simulink model "Quanser_AERO_Simulation_2020b"  (R2020b)
settings: Solver=ode45  StartTime=0.0  StopTime=sim_time  FixedStep=0.01  RelTol=1e-3
InitFcn:
  | % Run simulation parameters
  | quanser_AERO_sim_params;
model workspace (MAT data in the model file):
  a : Simulink.Parameter (value not decoded)
  a_a : Simulink.Parameter (value not decoded)
  b : Simulink.Parameter (value not decoded)
  b_b : Simulink.Parameter (value not decoded)
  c : Simulink.Parameter (value not decoded)
  c_c : Simulink.Parameter (value not decoded)
  d : Simulink.Parameter (value not decoded)
  d_d : Simulink.Parameter (value not decoded)
  e : Simulink.Parameter (value not decoded)
  f : Simulink.Parameter (value not decoded)
  g : Simulink.Parameter (value not decoded)
  p_p : Simulink.Parameter (value not decoded)
  smiData : object (value not decoded)
  t_t : Simulink.Parameter (value not decoded)
  u_lim : Simulink.Parameter (value not decoded)
  y_y : Simulink.Parameter (value not decoded)
  z_z : Simulink.Parameter (value not decoded)
values from neighbouring files (symbols this model uses):
  model = 2    [quanser_AERO_sim_params.m]
  ts = 0.002    [quanser_AERO_sim_params.m]
symbols that are objects in the model workspace (value not decoded): a, a_a, b, b_b, c, c_c, d, d_d, f, g, p_p, smiData, t_t, u_lim, y_y, z_z
undefined symbols (not defined in the file or in its folder): A, B, C, den1, den2, ini_cond, K, K_D1, K_D2, K_I1, K_I2, K_P1, K_P2, KI, KX, L, Nbar, noise, num1, num2, tau_p, X, Y, Z
libraries: sm_lib x175, nesl_utility x35, simulink x31
(part 5 of 5)

== system Quanser_AERO_Simulation_2020b/Quanser AERO3/Digital Twin/AERO_Base1_RIGID ==
  ReferenceFrame : sm_lib/Frames and Transforms/Reference Frame
  Solid : sm_lib/Body Elements/File Solid  ExtGeomFileName=AERO - Base_ipt_b1761deb.STEP  UnitType=FromFile  ExtGeomFileUnits=m  StepReaderType=HEX  ExportConvexHullGeometry=off  InertiaType=Custom  Mass=smiData.Solid(1).mass  MassUnits=kg  CenterOfMass=smiData.Solid(1).CoM  CenterOfMassUnits=mm  MomentsOfInertia=smiData.Solid(1).MoI  MomentsOfInertiaUnits=kg*mm^2  ProductsOfInertia=smiData.Solid(1).PoI  ProductsOfInertiaUnits=kg*mm^2  BasedOnType=DensityFromFile  Density=1000  DensityUnits=kg/m^3  DoExposeReferenceFrame=on  SerializedFrames=<Frames/>  GraphicType=FromGeometry  MarkerShape=Sphere  MarkerSize=10  GraphicVisPropType=SimpleVisualProperties  GraphicDiffuseColor=smiData.Solid(1).color  GraphicSpecularColor=[0.5 0.5 0.5 1.0]  GraphicAmbientColor=[0.15 0.15 0.15 1.0]  GraphicEmissiveColor=[0.0 0.0 0.0 1.0]  GraphicShininess=75  GraphicOpacity=smiData.Solid(1).opacity
  Transform : sm_lib/Frames and Transforms/Rigid Transform  TranslationMethod=Cartesian  TranslationStandardOffset=0  TranslationLengthUnit=mm  TranslationStandardAxis=+Z  TranslationCartesianOffset=smiData.RigidTransform(7).translation  TranslationROffset=0  TranslationROffsetUnits=m  TranslationZOffset=0  TranslationZOffsetUnits=m  TranslationThetaOffset=0  TranslationThetaOffsetUnits=deg  RotationMethod=ArbitraryAxis  RotationAngleUnits=rad  RotationStandardAxis=+Z  RotationAngle=smiData.RigidTransform(7).angle  RotationArbitraryAxis=smiData.RigidTransform(7).axis  FollAlignAxisA=+X  BaseAlignAxisA=+Y  FollAlignAxisB=+Y  BaseAlignAxisB=+Z  RotationSequenceAxes=FollowerAxes  RotationSequence=XYX  RotationSequenceAngles=[0 0 0]  RotationSequenceAnglesUnits=deg  RotationMatrix=[1 0 0; 0 1 0; 0 0 1]
  F1 : PMIOPort  Side=Left
  F : PMIOPort  Port=2  Side=Right
  connections:
  ReferenceFrame/RConn1 -- Solid/RConn1 -- Transform/LConn1 -- F1/RConn1
  Transform/RConn1 -- F/RConn1

== system Quanser_AERO_Simulation_2020b/Quanser AERO3/Digital Twin/AERO_Fork1_RIGID ==
  ReferenceFrame : sm_lib/Frames and Transforms/Reference Frame
  Solid : sm_lib/Body Elements/File Solid  ExtGeomFileName=AERO - Fork_ipt_cc713931.STEP  UnitType=FromFile  ExtGeomFileUnits=m  StepReaderType=HEX  ExportConvexHullGeometry=off  InertiaType=Custom  Mass=smiData.Solid(2).mass  MassUnits=kg  CenterOfMass=smiData.Solid(2).CoM  CenterOfMassUnits=mm  MomentsOfInertia=smiData.Solid(2).MoI  MomentsOfInertiaUnits=kg*mm^2  ProductsOfInertia=smiData.Solid(2).PoI  ProductsOfInertiaUnits=kg*mm^2  BasedOnType=DensityFromFile  Density=1000  DensityUnits=kg/m^3  DoExposeReferenceFrame=on  SerializedFrames=<Frames/>  GraphicType=FromGeometry  MarkerShape=Sphere  MarkerSize=10  GraphicVisPropType=SimpleVisualProperties  GraphicDiffuseColor=smiData.Solid(2).color  GraphicSpecularColor=[0.5 0.5 0.5 1.0]  GraphicAmbientColor=[0.15 0.15 0.15 1.0]  GraphicEmissiveColor=[0.0 0.0 0.0 1.0]  GraphicShininess=75  GraphicOpacity=smiData.Solid(2).opacity
  Transform : sm_lib/Frames and Transforms/Rigid Transform  TranslationMethod=Cartesian  TranslationStandardOffset=0  TranslationLengthUnit=mm  TranslationStandardAxis=+Z  TranslationCartesianOffset=smiData.RigidTransform(1).translation  TranslationROffset=0  TranslationROffsetUnits=m  TranslationZOffset=0  TranslationZOffsetUnits=m  TranslationThetaOffset=0  TranslationThetaOffsetUnits=deg  RotationMethod=ArbitraryAxis  RotationAngleUnits=rad  RotationStandardAxis=+Z  RotationAngle=smiData.RigidTransform(1).angle  RotationArbitraryAxis=smiData.RigidTransform(1).axis  FollAlignAxisA=+X  BaseAlignAxisA=+Y  FollAlignAxisB=+Y  BaseAlignAxisB=+Z  RotationSequenceAxes=FollowerAxes  RotationSequence=XYX  RotationSequenceAngles=[0 0 0]  RotationSequenceAnglesUnits=deg  RotationMatrix=[1 0 0; 0 1 0; 0 0 1]
  Transform1 : sm_lib/Frames and Transforms/Rigid Transform  TranslationMethod=Cartesian  TranslationStandardOffset=0  TranslationLengthUnit=mm  TranslationStandardAxis=+Z  TranslationCartesianOffset=smiData.RigidTransform(8).translation  TranslationROffset=0  TranslationROffsetUnits=m  TranslationZOffset=0  TranslationZOffsetUnits=m  TranslationThetaOffset=0  TranslationThetaOffsetUnits=deg  RotationMethod=ArbitraryAxis  RotationAngleUnits=rad  RotationStandardAxis=+Z  RotationAngle=smiData.RigidTransform(8).angle  RotationArbitraryAxis=smiData.RigidTransform(8).axis  FollAlignAxisA=+X  BaseAlignAxisA=+Y  FollAlignAxisB=+Y  BaseAlignAxisB=+Z  RotationSequenceAxes=FollowerAxes  RotationSequence=XYX  RotationSequenceAngles=[0 0 0]  RotationSequenceAnglesUnits=deg  RotationMatrix=[1 0 0; 0 1 0; 0 0 1]
  F1 : PMIOPort  Side=Left
  F : PMIOPort  Port=2  Side=Right
  connections:
  Transform/LConn1 -- Transform1/LConn1 -- ReferenceFrame/RConn1 -- Solid/RConn1
  Transform/RConn1 -- F/RConn1
  Transform1/RConn1 -- F1/RConn1

== system Quanser_AERO_Simulation_2020b/Quanser AERO3/Digital Twin/AERO_Propeller1_RIGID ==
  ReferenceFrame : sm_lib/Frames and Transforms/Reference Frame
  Solid : sm_lib/Body Elements/File Solid  ExtGeomFileName=AERO - Propeller_ipt_36a575e7.STEP  UnitType=FromFile  ExtGeomFileUnits=m  StepReaderType=HEX  ExportConvexHullGeometry=off  InertiaType=Custom  Mass=smiData.Solid(5).mass  MassUnits=kg  CenterOfMass=smiData.Solid(5).CoM  CenterOfMassUnits=mm  MomentsOfInertia=smiData.Solid(5).MoI  MomentsOfInertiaUnits=kg*mm^2  ProductsOfInertia=smiData.Solid(5).PoI  ProductsOfInertiaUnits=kg*mm^2  BasedOnType=DensityFromFile  Density=1000  DensityUnits=kg/m^3  DoExposeReferenceFrame=on  SerializedFrames=<Frames/>  GraphicType=FromGeometry  MarkerShape=Sphere  MarkerSize=10  GraphicVisPropType=SimpleVisualProperties  GraphicDiffuseColor=smiData.Solid(5).color  GraphicSpecularColor=[0.5 0.5 0.5 1.0]  GraphicAmbientColor=[0.15 0.15 0.15 1.0]  GraphicEmissiveColor=[0.0 0.0 0.0 1.0]  GraphicShininess=75  GraphicOpacity=smiData.Solid(5).opacity
  Transform : sm_lib/Frames and Transforms/Rigid Transform  TranslationMethod=Cartesian  TranslationStandardOffset=0  TranslationLengthUnit=mm  TranslationStandardAxis=+Z  TranslationCartesianOffset=smiData.RigidTransform(10).translation  TranslationROffset=0  TranslationROffsetUnits=m  TranslationZOffset=0  TranslationZOffsetUnits=m  TranslationThetaOffset=0  TranslationThetaOffsetUnits=deg  RotationMethod=ArbitraryAxis  RotationAngleUnits=rad  RotationStandardAxis=+Z  RotationAngle=smiData.RigidTransform(10).angle  RotationArbitraryAxis=smiData.RigidTransform(10).axis  FollAlignAxisA=+X  BaseAlignAxisA=+Y  FollAlignAxisB=+Y  BaseAlignAxisB=+Z  RotationSequenceAxes=FollowerAxes  RotationSequence=XYX  RotationSequenceAngles=[0 0 0]  RotationSequenceAnglesUnits=deg  RotationMatrix=[1 0 0; 0 1 0; 0 0 1]
  F : PMIOPort  Side=Left
  connections:
  ReferenceFrame/RConn1 -- Solid/RConn1 -- Transform/LConn1
  Transform/RConn1 -- F/RConn1

== system Quanser_AERO_Simulation_2020b/Quanser AERO3/Digital Twin/AERO_Propeller2_RIGID ==
  ReferenceFrame : sm_lib/Frames and Transforms/Reference Frame
  Solid : sm_lib/Body Elements/File Solid  ExtGeomFileName=AERO - Propeller_ipt_36a575e7.STEP  UnitType=FromFile  ExtGeomFileUnits=m  StepReaderType=HEX  ExportConvexHullGeometry=off  InertiaType=Custom  Mass=smiData.Solid(5).mass  MassUnits=kg  CenterOfMass=smiData.Solid(5).CoM  CenterOfMassUnits=mm  MomentsOfInertia=smiData.Solid(5).MoI  MomentsOfInertiaUnits=kg*mm^2  ProductsOfInertia=smiData.Solid(5).PoI  ProductsOfInertiaUnits=kg*mm^2  BasedOnType=DensityFromFile  Density=1000  DensityUnits=kg/m^3  DoExposeReferenceFrame=on  SerializedFrames=<Frames/>  GraphicType=FromGeometry  MarkerShape=Sphere  MarkerSize=10  GraphicVisPropType=SimpleVisualProperties  GraphicDiffuseColor=smiData.Solid(5).color  GraphicSpecularColor=[0.5 0.5 0.5 1.0]  GraphicAmbientColor=[0.15 0.15 0.15 1.0]  GraphicEmissiveColor=[0.0 0.0 0.0 1.0]  GraphicShininess=75  GraphicOpacity=smiData.Solid(5).opacity
  Transform : sm_lib/Frames and Transforms/Rigid Transform  TranslationMethod=Cartesian  TranslationStandardOffset=0  TranslationLengthUnit=mm  TranslationStandardAxis=+Z  TranslationCartesianOffset=smiData.RigidTransform(12).translation  TranslationROffset=0  TranslationROffsetUnits=m  TranslationZOffset=0  TranslationZOffsetUnits=m  TranslationThetaOffset=0  TranslationThetaOffsetUnits=deg  RotationMethod=ArbitraryAxis  RotationAngleUnits=rad  RotationStandardAxis=+Z  RotationAngle=smiData.RigidTransform(12).angle  RotationArbitraryAxis=smiData.RigidTransform(12).axis  FollAlignAxisA=+X  BaseAlignAxisA=+Y  FollAlignAxisB=+Y  BaseAlignAxisB=+Z  RotationSequenceAxes=FollowerAxes  RotationSequence=XYX  RotationSequenceAngles=[0 0 0]  RotationSequenceAnglesUnits=deg  RotationMatrix=[1 0 0; 0 1 0; 0 0 1]
  F : PMIOPort  Side=Left
  connections:
  ReferenceFrame/RConn1 -- Solid/RConn1 -- Transform/LConn1
  Transform/RConn1 -- F/RConn1

== system Quanser_AERO_Simulation_2020b/Quanser AERO3/Digital Twin/AERO_Propeller_Housing1_RIGID ==
  ReferenceFrame : sm_lib/Frames and Transforms/Reference Frame
  Solid : sm_lib/Body Elements/File Solid  ExtGeomFileName=AERO - Propeller Housing_ipt_f68ac60a.STEP  UnitType=FromFile  ExtGeomFileUnits=m  StepReaderType=HEX  ExportConvexHullGeometry=off  InertiaType=Custom  Mass=smiData.Solid(4).mass  MassUnits=kg  CenterOfMass=smiData.Solid(4).CoM  CenterOfMassUnits=mm  MomentsOfInertia=smiData.Solid(4).MoI  MomentsOfInertiaUnits=kg*mm^2  ProductsOfInertia=smiData.Solid(4).PoI  ProductsOfInertiaUnits=kg*mm^2  BasedOnType=DensityFromFile  Density=1000  DensityUnits=kg/m^3  DoExposeReferenceFrame=on  SerializedFrames=<Frames/>  GraphicType=FromGeometry  MarkerShape=Sphere  MarkerSize=10  GraphicVisPropType=SimpleVisualProperties  GraphicDiffuseColor=smiData.Solid(4).color  GraphicSpecularColor=[0.5 0.5 0.5 1.0]  GraphicAmbientColor=[0.15 0.15 0.15 1.0]  GraphicEmissiveColor=[0.0 0.0 0.0 1.0]  GraphicShininess=75  GraphicOpacity=smiData.Solid(4).opacity
  Transform : sm_lib/Frames and Transforms/Rigid Transform  TranslationMethod=Cartesian  TranslationStandardOffset=0  TranslationLengthUnit=mm  TranslationStandardAxis=+Z  TranslationCartesianOffset=smiData.RigidTransform(4).translation  TranslationROffset=0  TranslationROffsetUnits=m  TranslationZOffset=0  TranslationZOffsetUnits=m  TranslationThetaOffset=0  TranslationThetaOffsetUnits=deg  RotationMethod=ArbitraryAxis  RotationAngleUnits=rad  RotationStandardAxis=+Z  RotationAngle=smiData.RigidTransform(4).angle  RotationArbitraryAxis=smiData.RigidTransform(4).axis  FollAlignAxisA=+X  BaseAlignAxisA=+Y  FollAlignAxisB=+Y  BaseAlignAxisB=+Z  RotationSequenceAxes=FollowerAxes  RotationSequence=XYX  RotationSequenceAngles=[0 0 0]  RotationSequenceAnglesUnits=deg  RotationMatrix=[1 0 0; 0 1 0; 0 0 1]
  Transform1 : sm_lib/Frames and Transforms/Rigid Transform  TranslationMethod=Cartesian  TranslationStandardOffset=0  TranslationLengthUnit=mm  TranslationStandardAxis=+Z  TranslationCartesianOffset=smiData.RigidTransform(9).translation  TranslationROffset=0  TranslationROffsetUnits=m  TranslationZOffset=0  TranslationZOffsetUnits=m  TranslationThetaOffset=0  TranslationThetaOffsetUnits=deg  RotationMethod=ArbitraryAxis  RotationAngleUnits=rad  RotationStandardAxis=+Z  RotationAngle=smiData.RigidTransform(9).angle  RotationArbitraryAxis=smiData.RigidTransform(9).axis  FollAlignAxisA=+X  BaseAlignAxisA=+Y  FollAlignAxisB=+Y  BaseAlignAxisB=+Z  RotationSequenceAxes=FollowerAxes  RotationSequence=XYX  RotationSequenceAngles=[0 0 0]  RotationSequenceAnglesUnits=deg  RotationMatrix=[1 0 0; 0 1 0; 0 0 1]
  F : PMIOPort  Side=Left
  F1 : PMIOPort  Port=2  Side=Right
  connections:
  ReferenceFrame/RConn1 -- Solid/RConn1 -- Transform/LConn1 -- Transform1/LConn1
  Transform/RConn1 -- F/RConn1
  Transform1/RConn1 -- F1/RConn1

== system Quanser_AERO_Simulation_2020b/Quanser AERO3/Digital Twin/AERO_Propeller_Housing2_RIGID ==
  ReferenceFrame : sm_lib/Frames and Transforms/Reference Frame
  Solid : sm_lib/Body Elements/File Solid  ExtGeomFileName=AERO - Propeller Housing_ipt_f68ac60a.STEP  UnitType=FromFile  ExtGeomFileUnits=m  StepReaderType=HEX  ExportConvexHullGeometry=off  InertiaType=Custom  Mass=smiData.Solid(4).mass  MassUnits=kg  CenterOfMass=smiData.Solid(4).CoM  CenterOfMassUnits=mm  MomentsOfInertia=smiData.Solid(4).MoI  MomentsOfInertiaUnits=kg*mm^2  ProductsOfInertia=smiData.Solid(4).PoI  ProductsOfInertiaUnits=kg*mm^2  BasedOnType=DensityFromFile  Density=1000  DensityUnits=kg/m^3  DoExposeReferenceFrame=on  SerializedFrames=<Frames/>  GraphicType=FromGeometry  MarkerShape=Sphere  MarkerSize=10  GraphicVisPropType=SimpleVisualProperties  GraphicDiffuseColor=smiData.Solid(4).color  GraphicSpecularColor=[0.5 0.5 0.5 1.0]  GraphicAmbientColor=[0.15 0.15 0.15 1.0]  GraphicEmissiveColor=[0.0 0.0 0.0 1.0]  GraphicShininess=75  GraphicOpacity=smiData.Solid(4).opacity
  Transform : sm_lib/Frames and Transforms/Rigid Transform  TranslationMethod=Cartesian  TranslationStandardOffset=0  TranslationLengthUnit=mm  TranslationStandardAxis=+Z  TranslationCartesianOffset=smiData.RigidTransform(6).translation  TranslationROffset=0  TranslationROffsetUnits=m  TranslationZOffset=0  TranslationZOffsetUnits=m  TranslationThetaOffset=0  TranslationThetaOffsetUnits=deg  RotationMethod=ArbitraryAxis  RotationAngleUnits=rad  RotationStandardAxis=+Z  RotationAngle=smiData.RigidTransform(6).angle  RotationArbitraryAxis=smiData.RigidTransform(6).axis  FollAlignAxisA=+X  BaseAlignAxisA=+Y  FollAlignAxisB=+Y  BaseAlignAxisB=+Z  RotationSequenceAxes=FollowerAxes  RotationSequence=XYX  RotationSequenceAngles=[0 0 0]  RotationSequenceAnglesUnits=deg  RotationMatrix=[1 0 0; 0 1 0; 0 0 1]
  Transform1 : sm_lib/Frames and Transforms/Rigid Transform  TranslationMethod=Cartesian  TranslationStandardOffset=0  TranslationLengthUnit=mm  TranslationStandardAxis=+Z  TranslationCartesianOffset=smiData.RigidTransform(11).translation  TranslationROffset=0  TranslationROffsetUnits=m  TranslationZOffset=0  TranslationZOffsetUnits=m  TranslationThetaOffset=0  TranslationThetaOffsetUnits=deg  RotationMethod=ArbitraryAxis  RotationAngleUnits=rad  RotationStandardAxis=+Z  RotationAngle=smiData.RigidTransform(11).angle  RotationArbitraryAxis=smiData.RigidTransform(11).axis  FollAlignAxisA=+X  BaseAlignAxisA=+Y  FollAlignAxisB=+Y  BaseAlignAxisB=+Z  RotationSequenceAxes=FollowerAxes  RotationSequence=XYX  RotationSequenceAngles=[0 0 0]  RotationSequenceAnglesUnits=deg  RotationMatrix=[1 0 0; 0 1 0; 0 0 1]
  F : PMIOPort  Side=Left
  F1 : PMIOPort  Port=2  Side=Right
  connections:
  ReferenceFrame/RConn1 -- Solid/RConn1 -- Transform/LConn1 -- Transform1/LConn1
  Transform/RConn1 -- F/RConn1
  Transform1/RConn1 -- F1/RConn1

== system Quanser_AERO_Simulation_2020b/Quanser AERO4/Digital Twin/AERO_Arm1_RIGID ==
  ReferenceFrame : sm_lib/Frames and Transforms/Reference Frame
  Solid : sm_lib/Body Elements/File Solid  ExtGeomFileName=AERO - Arm_ipt_54056d2d.STEP  UnitType=FromFile  ExtGeomFileUnits=m  StepReaderType=HEX  ExportConvexHullGeometry=off  InertiaType=Custom  Mass=smiData.Solid(3).mass  MassUnits=kg  CenterOfMass=smiData.Solid(3).CoM  CenterOfMassUnits=mm  MomentsOfInertia=smiData.Solid(3).MoI  MomentsOfInertiaUnits=kg*mm^2  ProductsOfInertia=smiData.Solid(3).PoI  ProductsOfInertiaUnits=kg*mm^2  BasedOnType=DensityFromFile  Density=1000  DensityUnits=kg/m^3  DoExposeReferenceFrame=on  SerializedFrames=<Frames/>  GraphicType=FromGeometry  MarkerShape=Sphere  MarkerSize=10  GraphicVisPropType=SimpleVisualProperties  GraphicDiffuseColor=smiData.Solid(3).color  GraphicSpecularColor=[0.5 0.5 0.5 1.0]  GraphicAmbientColor=[0.15 0.15 0.15 1.0]  GraphicEmissiveColor=[0.0 0.0 0.0 1.0]  GraphicShininess=75  GraphicOpacity=smiData.Solid(3).opacity
  Transform : sm_lib/Frames and Transforms/Rigid Transform  TranslationMethod=Cartesian  TranslationStandardOffset=0  TranslationLengthUnit=mm  TranslationStandardAxis=+Z  TranslationCartesianOffset=smiData.RigidTransform(2).translation  TranslationROffset=0  TranslationROffsetUnits=m  TranslationZOffset=0  TranslationZOffsetUnits=m  TranslationThetaOffset=0  TranslationThetaOffsetUnits=deg  RotationMethod=ArbitraryAxis  RotationAngleUnits=rad  RotationStandardAxis=+Z  RotationAngle=smiData.RigidTransform(2).angle  RotationArbitraryAxis=smiData.RigidTransform(2).axis  FollAlignAxisA=+X  BaseAlignAxisA=+Y  FollAlignAxisB=+Y  BaseAlignAxisB=+Z  RotationSequenceAxes=FollowerAxes  RotationSequence=XYX  RotationSequenceAngles=[0 0 0]  RotationSequenceAnglesUnits=deg  RotationMatrix=[1 0 0; 0 1 0; 0 0 1]
  Transform1 : sm_lib/Frames and Transforms/Rigid Transform  TranslationMethod=Cartesian  TranslationStandardOffset=0  TranslationLengthUnit=mm  TranslationStandardAxis=+Z  TranslationCartesianOffset=smiData.RigidTransform(3).translation  TranslationROffset=0  TranslationROffsetUnits=m  TranslationZOffset=0  TranslationZOffsetUnits=m  TranslationThetaOffset=0  TranslationThetaOffsetUnits=deg  RotationMethod=ArbitraryAxis  RotationAngleUnits=rad  RotationStandardAxis=+Z  RotationAngle=smiData.RigidTransform(3).angle  RotationArbitraryAxis=smiData.RigidTransform(3).axis  FollAlignAxisA=+X  BaseAlignAxisA=+Y  FollAlignAxisB=+Y  BaseAlignAxisB=+Z  RotationSequenceAxes=FollowerAxes  RotationSequence=XYX  RotationSequenceAngles=[0 0 0]  RotationSequenceAnglesUnits=deg  RotationMatrix=[1 0 0; 0 1 0; 0 0 1]
  Transform2 : sm_lib/Frames and Transforms/Rigid Transform  TranslationMethod=Cartesian  TranslationStandardOffset=0  TranslationLengthUnit=mm  TranslationStandardAxis=+Z  TranslationCartesianOffset=smiData.RigidTransform(5).translation  TranslationROffset=0  TranslationROffsetUnits=m  TranslationZOffset=0  TranslationZOffsetUnits=m  TranslationThetaOffset=0  TranslationThetaOffsetUnits=deg  RotationMethod=ArbitraryAxis  RotationAngleUnits=rad  RotationStandardAxis=+Z  RotationAngle=smiData.RigidTransform(5).angle  RotationArbitraryAxis=smiData.RigidTransform(5).axis  FollAlignAxisA=+X  BaseAlignAxisA=+Y  FollAlignAxisB=+Y  BaseAlignAxisB=+Z  RotationSequenceAxes=FollowerAxes  RotationSequence=XYX  RotationSequenceAngles=[0 0 0]  RotationSequenceAnglesUnits=deg  RotationMatrix=[1 0 0; 0 1 0; 0 0 1]
  F : PMIOPort  Side=Left
  F2 : PMIOPort  Port=2  Side=Right
  F1 : PMIOPort  Port=3  Side=Right
  connections:
  Transform1/LConn1 -- Transform2/LConn1 -- ReferenceFrame/RConn1 -- Solid/RConn1 -- Transform/LConn1
  Transform/RConn1 -- F/RConn1
  Transform1/RConn1 -- F1/RConn1
  Transform2/RConn1 -- F2/RConn1

== system Quanser_AERO_Simulation_2020b/Quanser AERO4/Digital Twin/AERO_Base1_RIGID ==
  ReferenceFrame : sm_lib/Frames and Transforms/Reference Frame
  Solid : sm_lib/Body Elements/File Solid  ExtGeomFileName=AERO - Base_ipt_b1761deb.STEP  UnitType=FromFile  ExtGeomFileUnits=m  StepReaderType=HEX  ExportConvexHullGeometry=off  InertiaType=Custom  Mass=smiData.Solid(1).mass  MassUnits=kg  CenterOfMass=smiData.Solid(1).CoM  CenterOfMassUnits=mm  MomentsOfInertia=smiData.Solid(1).MoI  MomentsOfInertiaUnits=kg*mm^2  ProductsOfInertia=smiData.Solid(1).PoI  ProductsOfInertiaUnits=kg*mm^2  BasedOnType=DensityFromFile  Density=1000  DensityUnits=kg/m^3  DoExposeReferenceFrame=on  SerializedFrames=<Frames/>  GraphicType=FromGeometry  MarkerShape=Sphere  MarkerSize=10  GraphicVisPropType=SimpleVisualProperties  GraphicDiffuseColor=smiData.Solid(1).color  GraphicSpecularColor=[0.5 0.5 0.5 1.0]  GraphicAmbientColor=[0.15 0.15 0.15 1.0]  GraphicEmissiveColor=[0.0 0.0 0.0 1.0]  GraphicShininess=75  GraphicOpacity=smiData.Solid(1).opacity
  Transform : sm_lib/Frames and Transforms/Rigid Transform  TranslationMethod=Cartesian  TranslationStandardOffset=0  TranslationLengthUnit=mm  TranslationStandardAxis=+Z  TranslationCartesianOffset=smiData.RigidTransform(7).translation  TranslationROffset=0  TranslationROffsetUnits=m  TranslationZOffset=0  TranslationZOffsetUnits=m  TranslationThetaOffset=0  TranslationThetaOffsetUnits=deg  RotationMethod=ArbitraryAxis  RotationAngleUnits=rad  RotationStandardAxis=+Z  RotationAngle=smiData.RigidTransform(7).angle  RotationArbitraryAxis=smiData.RigidTransform(7).axis  FollAlignAxisA=+X  BaseAlignAxisA=+Y  FollAlignAxisB=+Y  BaseAlignAxisB=+Z  RotationSequenceAxes=FollowerAxes  RotationSequence=XYX  RotationSequenceAngles=[0 0 0]  RotationSequenceAnglesUnits=deg  RotationMatrix=[1 0 0; 0 1 0; 0 0 1]
  F1 : PMIOPort  Side=Left
  F : PMIOPort  Port=2  Side=Right
  connections:
  ReferenceFrame/RConn1 -- Solid/RConn1 -- Transform/LConn1 -- F1/RConn1
  Transform/RConn1 -- F/RConn1

== system Quanser_AERO_Simulation_2020b/Quanser AERO4/Digital Twin/AERO_Fork1_RIGID ==
  ReferenceFrame : sm_lib/Frames and Transforms/Reference Frame
  Solid : sm_lib/Body Elements/File Solid  ExtGeomFileName=AERO - Fork_ipt_cc713931.STEP  UnitType=FromFile  ExtGeomFileUnits=m  StepReaderType=HEX  ExportConvexHullGeometry=off  InertiaType=Custom  Mass=smiData.Solid(2).mass  MassUnits=kg  CenterOfMass=smiData.Solid(2).CoM  CenterOfMassUnits=mm  MomentsOfInertia=smiData.Solid(2).MoI  MomentsOfInertiaUnits=kg*mm^2  ProductsOfInertia=smiData.Solid(2).PoI  ProductsOfInertiaUnits=kg*mm^2  BasedOnType=DensityFromFile  Density=1000  DensityUnits=kg/m^3  DoExposeReferenceFrame=on  SerializedFrames=<Frames/>  GraphicType=FromGeometry  MarkerShape=Sphere  MarkerSize=10  GraphicVisPropType=SimpleVisualProperties  GraphicDiffuseColor=smiData.Solid(2).color  GraphicSpecularColor=[0.5 0.5 0.5 1.0]  GraphicAmbientColor=[0.15 0.15 0.15 1.0]  GraphicEmissiveColor=[0.0 0.0 0.0 1.0]  GraphicShininess=75  GraphicOpacity=smiData.Solid(2).opacity
  Transform : sm_lib/Frames and Transforms/Rigid Transform  TranslationMethod=Cartesian  TranslationStandardOffset=0  TranslationLengthUnit=mm  TranslationStandardAxis=+Z  TranslationCartesianOffset=smiData.RigidTransform(1).translation  TranslationROffset=0  TranslationROffsetUnits=m  TranslationZOffset=0  TranslationZOffsetUnits=m  TranslationThetaOffset=0  TranslationThetaOffsetUnits=deg  RotationMethod=ArbitraryAxis  RotationAngleUnits=rad  RotationStandardAxis=+Z  RotationAngle=smiData.RigidTransform(1).angle  RotationArbitraryAxis=smiData.RigidTransform(1).axis  FollAlignAxisA=+X  BaseAlignAxisA=+Y  FollAlignAxisB=+Y  BaseAlignAxisB=+Z  RotationSequenceAxes=FollowerAxes  RotationSequence=XYX  RotationSequenceAngles=[0 0 0]  RotationSequenceAnglesUnits=deg  RotationMatrix=[1 0 0; 0 1 0; 0 0 1]
  Transform1 : sm_lib/Frames and Transforms/Rigid Transform  TranslationMethod=Cartesian  TranslationStandardOffset=0  TranslationLengthUnit=mm  TranslationStandardAxis=+Z  TranslationCartesianOffset=smiData.RigidTransform(8).translation  TranslationROffset=0  TranslationROffsetUnits=m  TranslationZOffset=0  TranslationZOffsetUnits=m  TranslationThetaOffset=0  TranslationThetaOffsetUnits=deg  RotationMethod=ArbitraryAxis  RotationAngleUnits=rad  RotationStandardAxis=+Z  RotationAngle=smiData.RigidTransform(8).angle  RotationArbitraryAxis=smiData.RigidTransform(8).axis  FollAlignAxisA=+X  BaseAlignAxisA=+Y  FollAlignAxisB=+Y  BaseAlignAxisB=+Z  RotationSequenceAxes=FollowerAxes  RotationSequence=XYX  RotationSequenceAngles=[0 0 0]  RotationSequenceAnglesUnits=deg  RotationMatrix=[1 0 0; 0 1 0; 0 0 1]
  F1 : PMIOPort  Side=Left
  F : PMIOPort  Port=2  Side=Right
  connections:
  Transform/LConn1 -- Transform1/LConn1 -- ReferenceFrame/RConn1 -- Solid/RConn1
  Transform/RConn1 -- F/RConn1
  Transform1/RConn1 -- F1/RConn1

== system Quanser_AERO_Simulation_2020b/Quanser AERO4/Digital Twin/AERO_Propeller1_RIGID ==
  ReferenceFrame : sm_lib/Frames and Transforms/Reference Frame
  Solid : sm_lib/Body Elements/File Solid  ExtGeomFileName=AERO - Propeller_ipt_36a575e7.STEP  UnitType=FromFile  ExtGeomFileUnits=m  StepReaderType=HEX  ExportConvexHullGeometry=off  InertiaType=Custom  Mass=smiData.Solid(5).mass  MassUnits=kg  CenterOfMass=smiData.Solid(5).CoM  CenterOfMassUnits=mm  MomentsOfInertia=smiData.Solid(5).MoI  MomentsOfInertiaUnits=kg*mm^2  ProductsOfInertia=smiData.Solid(5).PoI  ProductsOfInertiaUnits=kg*mm^2  BasedOnType=DensityFromFile  Density=1000  DensityUnits=kg/m^3  DoExposeReferenceFrame=on  SerializedFrames=<Frames/>  GraphicType=FromGeometry  MarkerShape=Sphere  MarkerSize=10  GraphicVisPropType=SimpleVisualProperties  GraphicDiffuseColor=smiData.Solid(5).color  GraphicSpecularColor=[0.5 0.5 0.5 1.0]  GraphicAmbientColor=[0.15 0.15 0.15 1.0]  GraphicEmissiveColor=[0.0 0.0 0.0 1.0]  GraphicShininess=75  GraphicOpacity=smiData.Solid(5).opacity
  Transform : sm_lib/Frames and Transforms/Rigid Transform  TranslationMethod=Cartesian  TranslationStandardOffset=0  TranslationLengthUnit=mm  TranslationStandardAxis=+Z  TranslationCartesianOffset=smiData.RigidTransform(10).translation  TranslationROffset=0  TranslationROffsetUnits=m  TranslationZOffset=0  TranslationZOffsetUnits=m  TranslationThetaOffset=0  TranslationThetaOffsetUnits=deg  RotationMethod=ArbitraryAxis  RotationAngleUnits=rad  RotationStandardAxis=+Z  RotationAngle=smiData.RigidTransform(10).angle  RotationArbitraryAxis=smiData.RigidTransform(10).axis  FollAlignAxisA=+X  BaseAlignAxisA=+Y  FollAlignAxisB=+Y  BaseAlignAxisB=+Z  RotationSequenceAxes=FollowerAxes  RotationSequence=XYX  RotationSequenceAngles=[0 0 0]  RotationSequenceAnglesUnits=deg  RotationMatrix=[1 0 0; 0 1 0; 0 0 1]
  F : PMIOPort  Side=Left
  connections:
  ReferenceFrame/RConn1 -- Solid/RConn1 -- Transform/LConn1
  Transform/RConn1 -- F/RConn1

== system Quanser_AERO_Simulation_2020b/Quanser AERO4/Digital Twin/AERO_Propeller2_RIGID ==
  ReferenceFrame : sm_lib/Frames and Transforms/Reference Frame
  Solid : sm_lib/Body Elements/File Solid  ExtGeomFileName=AERO - Propeller_ipt_36a575e7.STEP  UnitType=FromFile  ExtGeomFileUnits=m  StepReaderType=HEX  ExportConvexHullGeometry=off  InertiaType=Custom  Mass=smiData.Solid(5).mass  MassUnits=kg  CenterOfMass=smiData.Solid(5).CoM  CenterOfMassUnits=mm  MomentsOfInertia=smiData.Solid(5).MoI  MomentsOfInertiaUnits=kg*mm^2  ProductsOfInertia=smiData.Solid(5).PoI  ProductsOfInertiaUnits=kg*mm^2  BasedOnType=DensityFromFile  Density=1000  DensityUnits=kg/m^3  DoExposeReferenceFrame=on  SerializedFrames=<Frames/>  GraphicType=FromGeometry  MarkerShape=Sphere  MarkerSize=10  GraphicVisPropType=SimpleVisualProperties  GraphicDiffuseColor=smiData.Solid(5).color  GraphicSpecularColor=[0.5 0.5 0.5 1.0]  GraphicAmbientColor=[0.15 0.15 0.15 1.0]  GraphicEmissiveColor=[0.0 0.0 0.0 1.0]  GraphicShininess=75  GraphicOpacity=smiData.Solid(5).opacity
  Transform : sm_lib/Frames and Transforms/Rigid Transform  TranslationMethod=Cartesian  TranslationStandardOffset=0  TranslationLengthUnit=mm  TranslationStandardAxis=+Z  TranslationCartesianOffset=smiData.RigidTransform(12).translation  TranslationROffset=0  TranslationROffsetUnits=m  TranslationZOffset=0  TranslationZOffsetUnits=m  TranslationThetaOffset=0  TranslationThetaOffsetUnits=deg  RotationMethod=ArbitraryAxis  RotationAngleUnits=rad  RotationStandardAxis=+Z  RotationAngle=smiData.RigidTransform(12).angle  RotationArbitraryAxis=smiData.RigidTransform(12).axis  FollAlignAxisA=+X  BaseAlignAxisA=+Y  FollAlignAxisB=+Y  BaseAlignAxisB=+Z  RotationSequenceAxes=FollowerAxes  RotationSequence=XYX  RotationSequenceAngles=[0 0 0]  RotationSequenceAnglesUnits=deg  RotationMatrix=[1 0 0; 0 1 0; 0 0 1]
  F : PMIOPort  Side=Left
  connections:
  ReferenceFrame/RConn1 -- Solid/RConn1 -- Transform/LConn1
  Transform/RConn1 -- F/RConn1

== system Quanser_AERO_Simulation_2020b/Quanser AERO4/Digital Twin/AERO_Propeller_Housing1_RIGID ==
  ReferenceFrame : sm_lib/Frames and Transforms/Reference Frame
  Solid : sm_lib/Body Elements/File Solid  ExtGeomFileName=AERO - Propeller Housing_ipt_f68ac60a.STEP  UnitType=FromFile  ExtGeomFileUnits=m  StepReaderType=HEX  ExportConvexHullGeometry=off  InertiaType=Custom  Mass=smiData.Solid(4).mass  MassUnits=kg  CenterOfMass=smiData.Solid(4).CoM  CenterOfMassUnits=mm  MomentsOfInertia=smiData.Solid(4).MoI  MomentsOfInertiaUnits=kg*mm^2  ProductsOfInertia=smiData.Solid(4).PoI  ProductsOfInertiaUnits=kg*mm^2  BasedOnType=DensityFromFile  Density=1000  DensityUnits=kg/m^3  DoExposeReferenceFrame=on  SerializedFrames=<Frames/>  GraphicType=FromGeometry  MarkerShape=Sphere  MarkerSize=10  GraphicVisPropType=SimpleVisualProperties  GraphicDiffuseColor=smiData.Solid(4).color  GraphicSpecularColor=[0.5 0.5 0.5 1.0]  GraphicAmbientColor=[0.15 0.15 0.15 1.0]  GraphicEmissiveColor=[0.0 0.0 0.0 1.0]  GraphicShininess=75  GraphicOpacity=smiData.Solid(4).opacity
  Transform : sm_lib/Frames and Transforms/Rigid Transform  TranslationMethod=Cartesian  TranslationStandardOffset=0  TranslationLengthUnit=mm  TranslationStandardAxis=+Z  TranslationCartesianOffset=smiData.RigidTransform(4).translation  TranslationROffset=0  TranslationROffsetUnits=m  TranslationZOffset=0  TranslationZOffsetUnits=m  TranslationThetaOffset=0  TranslationThetaOffsetUnits=deg  RotationMethod=ArbitraryAxis  RotationAngleUnits=rad  RotationStandardAxis=+Z  RotationAngle=smiData.RigidTransform(4).angle  RotationArbitraryAxis=smiData.RigidTransform(4).axis  FollAlignAxisA=+X  BaseAlignAxisA=+Y  FollAlignAxisB=+Y  BaseAlignAxisB=+Z  RotationSequenceAxes=FollowerAxes  RotationSequence=XYX  RotationSequenceAngles=[0 0 0]  RotationSequenceAnglesUnits=deg  RotationMatrix=[1 0 0; 0 1 0; 0 0 1]
  Transform1 : sm_lib/Frames and Transforms/Rigid Transform  TranslationMethod=Cartesian  TranslationStandardOffset=0  TranslationLengthUnit=mm  TranslationStandardAxis=+Z  TranslationCartesianOffset=smiData.RigidTransform(9).translation  TranslationROffset=0  TranslationROffsetUnits=m  TranslationZOffset=0  TranslationZOffsetUnits=m  TranslationThetaOffset=0  TranslationThetaOffsetUnits=deg  RotationMethod=ArbitraryAxis  RotationAngleUnits=rad  RotationStandardAxis=+Z  RotationAngle=smiData.RigidTransform(9).angle  RotationArbitraryAxis=smiData.RigidTransform(9).axis  FollAlignAxisA=+X  BaseAlignAxisA=+Y  FollAlignAxisB=+Y  BaseAlignAxisB=+Z  RotationSequenceAxes=FollowerAxes  RotationSequence=XYX  RotationSequenceAngles=[0 0 0]  RotationSequenceAnglesUnits=deg  RotationMatrix=[1 0 0; 0 1 0; 0 0 1]
  F : PMIOPort  Side=Left
  F1 : PMIOPort  Port=2  Side=Right
  connections:
  ReferenceFrame/RConn1 -- Solid/RConn1 -- Transform/LConn1 -- Transform1/LConn1
  Transform/RConn1 -- F/RConn1
  Transform1/RConn1 -- F1/RConn1

== system Quanser_AERO_Simulation_2020b/Quanser AERO4/Digital Twin/AERO_Propeller_Housing2_RIGID ==
  ReferenceFrame : sm_lib/Frames and Transforms/Reference Frame
  Solid : sm_lib/Body Elements/File Solid  ExtGeomFileName=AERO - Propeller Housing_ipt_f68ac60a.STEP  UnitType=FromFile  ExtGeomFileUnits=m  StepReaderType=HEX  ExportConvexHullGeometry=off  InertiaType=Custom  Mass=smiData.Solid(4).mass  MassUnits=kg  CenterOfMass=smiData.Solid(4).CoM  CenterOfMassUnits=mm  MomentsOfInertia=smiData.Solid(4).MoI  MomentsOfInertiaUnits=kg*mm^2  ProductsOfInertia=smiData.Solid(4).PoI  ProductsOfInertiaUnits=kg*mm^2  BasedOnType=DensityFromFile  Density=1000  DensityUnits=kg/m^3  DoExposeReferenceFrame=on  SerializedFrames=<Frames/>  GraphicType=FromGeometry  MarkerShape=Sphere  MarkerSize=10  GraphicVisPropType=SimpleVisualProperties  GraphicDiffuseColor=smiData.Solid(4).color  GraphicSpecularColor=[0.5 0.5 0.5 1.0]  GraphicAmbientColor=[0.15 0.15 0.15 1.0]  GraphicEmissiveColor=[0.0 0.0 0.0 1.0]  GraphicShininess=75  GraphicOpacity=smiData.Solid(4).opacity
  Transform : sm_lib/Frames and Transforms/Rigid Transform  TranslationMethod=Cartesian  TranslationStandardOffset=0  TranslationLengthUnit=mm  TranslationStandardAxis=+Z  TranslationCartesianOffset=smiData.RigidTransform(6).translation  TranslationROffset=0  TranslationROffsetUnits=m  TranslationZOffset=0  TranslationZOffsetUnits=m  TranslationThetaOffset=0  TranslationThetaOffsetUnits=deg  RotationMethod=ArbitraryAxis  RotationAngleUnits=rad  RotationStandardAxis=+Z  RotationAngle=smiData.RigidTransform(6).angle  RotationArbitraryAxis=smiData.RigidTransform(6).axis  FollAlignAxisA=+X  BaseAlignAxisA=+Y  FollAlignAxisB=+Y  BaseAlignAxisB=+Z  RotationSequenceAxes=FollowerAxes  RotationSequence=XYX  RotationSequenceAngles=[0 0 0]  RotationSequenceAnglesUnits=deg  RotationMatrix=[1 0 0; 0 1 0; 0 0 1]
  Transform1 : sm_lib/Frames and Transforms/Rigid Transform  TranslationMethod=Cartesian  TranslationStandardOffset=0  TranslationLengthUnit=mm  TranslationStandardAxis=+Z  TranslationCartesianOffset=smiData.RigidTransform(11).translation  TranslationROffset=0  TranslationROffsetUnits=m  TranslationZOffset=0  TranslationZOffsetUnits=m  TranslationThetaOffset=0  TranslationThetaOffsetUnits=deg  RotationMethod=ArbitraryAxis  RotationAngleUnits=rad  RotationStandardAxis=+Z  RotationAngle=smiData.RigidTransform(11).angle  RotationArbitraryAxis=smiData.RigidTransform(11).axis  FollAlignAxisA=+X  BaseAlignAxisA=+Y  FollAlignAxisB=+Y  BaseAlignAxisB=+Z  RotationSequenceAxes=FollowerAxes  RotationSequence=XYX  RotationSequenceAngles=[0 0 0]  RotationSequenceAnglesUnits=deg  RotationMatrix=[1 0 0; 0 1 0; 0 0 1]
  F : PMIOPort  Side=Left
  F1 : PMIOPort  Port=2  Side=Right
  connections:
  ReferenceFrame/RConn1 -- Solid/RConn1 -- Transform/LConn1 -- Transform1/LConn1
  Transform/RConn1 -- F/RConn1
  Transform1/RConn1 -- F1/RConn1

== matlab function Quanser_AERO_Simulation_2020b/Quanser AERO1/Quanser AERO System Dynamics/MATLAB Function ==
  data: x input; u input; x_dot output; model input; a parameter; b parameter; c parameter; d parameter; e parameter; f parameter; g parameter; a_a parameter; b_b parameter; c_c parameter; d_d parameter; p_p parameter; t_t parameter; y_y parameter; z_z parameter
% ============================================================= %
%    This function computes the dynamics for the Quanser AERO   %
%    It takes the current input u = (V0, V1), the current       %
%    state x = (theta, theta_dot, psi, psi_dot) and the model   %
%    configuration ("1DOF": 1 or "2DOF": 2) and outputs x_dot   %
%    Created by Vincent Liu (liuv2@student.unimelb.edu.au)      %
%    For ELEN90064 Advanced Control Systems Workshops           %
%    Last updated: 29-07-21                                     %
% ============================================================= %

function x_dot = get_x_dot(x, u, model, a, b, c, d, e, f, g, a_a, b_b, c_c, d_d, p_p, t_t, y_y, z_z)

if (model == 1)
    tau_b_f_0 = 0.8*d;
else
    tau_b_f_0 = 0.8*p_p;
end
tau_b_f_1 = t_t;

eps = 1e-8;

p = x(1); q = x(2); n = x(3); m = x(4);
r = u(1); t = u(2);

q_dot = 0.0;
m_dot = 0.0;
tau_f_0 = 0;

if (abs(q) > eps)
    tau_f_0 = tau_b_f_0*sign(q);
else
    tau_f_0 = 0;
end

if (abs(m) > eps)
    tau_f_1 = tau_b_f_1*sign(m);
else
    tau_f_1 = 0;
end

if (model == 1)
    q_dot = (1/b)*(d*r - tau_f_0 - a_a*q - c*sin(p));
    m_dot = 0;
else
    q_dot =  -(tau_f_0*z_z + b_b*q*z_z - p_p*r*z_z + a*d_d^2*tau_f_0 - f*t*t_t*z_z + a*e^2*tau_f_0*sin(p)^2 + a*b_b*d_d^2*q - a*d_d^2*p_p*r + a^2*e^3*g*sin(p)^3 + a^2*d_d^2*e*g*sin(p) + a*b_b*e^2*q*sin(p)^2 - a*e^2*p_p*r*sin(p)^2 - a^2*e^4*m^2*cos(p)*sin(p)^3 + a*d_d*e*tau_f_1*cos(p) - a*d_d^2*f*t*t_t + a*e*g*z_z*sin(p) - a*e^2*f*t*t_t*sin(p)^2 - a^2*d_d^2*e^2*m^2*cos(p)*sin(p) + a*c_c*d_d*e*m*cos(p) + a^2*d_d^2*e^2*q^2*cos(p)*sin(p) - a*d_d*e*t*t_t*cos(p) - a*e^2*m^2*z_z*cos(p)*sin(p) + 2*a^2*d_d*e^3*m*q*cos(p)^2*sin(p) - a*d_d*e*f*p_p*r*cos(p))/(- a^2*d_d^2*e^2*cos(p)^2 + a^2*d_d^2*e^2 + a^2*e^4*sin(p)^2 + y_y*a*d_d^2 + y_y*a*e^2*sin(p)^2 + z_z*a*e^2 + y_y*z_z);
    m_dot = -(tau_f_1*y_y + c_c*m*y_y - t*t_t*y_y + a*e^2*tau_f_1 - f*p_p*r*y_y + a*c_c*e^2*m - a*e^2*t*t_t - a*e^2*f*p_p*r + a*d_d*e*tau_f_0*cos(p) + a^2*d_d*e^3*q^2*sin(p) - a^2*d_d*e^3*m^2*cos(p)^2*sin(p) + a*b_b*d_d*e*q*cos(p) - a*d_d*e*p_p*r*cos(p) + a^2*d_d*e^2*g*cos(p)*sin(p) + 2*a^2*e^4*m*q*cos(p)*sin(p) + a*d_d*e*q^2*y_y*sin(p) + 2*a*e^2*m*q*y_y*cos(p)*sin(p) - a*d_d*e*f*t*t_t*cos(p))/(- a^2*d_d^2*e^2*cos(p)^2 + a^2*d_d^2*e^2 + a^2*e^4*sin(p)^2 + y_y*a*d_d^2 + y_y*a*e^2*sin(p)^2 + z_z*a*e^2 + y_y*z_z);
end

x_dot = [q; q_dot; m; m_dot];

end

== matlab function Quanser_AERO_Simulation_2020b/Quanser AERO2/Quanser AERO System Dynamics/MATLAB Function ==
  data: x input; u input; x_dot output; model input; a parameter; b parameter; c parameter; d parameter; e parameter; f parameter; g parameter; a_a parameter; b_b parameter; c_c parameter; d_d parameter; p_p parameter; t_t parameter; y_y parameter; z_z parameter
% ============================================================= %
%    This function computes the dynamics for the Quanser AERO   %
%    It takes the current input u = (V0, V1), the current       %
%    state x = (theta, theta_dot, psi, psi_dot) and the model   %
%    configuration ("1DOF": 1 or "2DOF": 2) and outputs x_dot   %
%    Created by Vincent Liu (liuv2@student.unimelb.edu.au)      %
%    For ELEN90064 Advanced Control Systems Workshops           %
%    Last updated: 29-07-21                                     %
% ============================================================= %

function x_dot = get_x_dot(x, u, model, a, b, c, d, e, f, g, a_a, b_b, c_c, d_d, p_p, t_t, y_y, z_z)

if (model == 1)
    tau_b_f_0 = 0.8*d;
else
    tau_b_f_0 = 0.8*p_p;
end
tau_b_f_1 = t_t;

eps = 1e-8;

p = x(1); q = x(2); n = x(3); m = x(4);
r = u(1); t = u(2);

q_dot = 0.0;
m_dot = 0.0;
tau_f_0 = 0;

if (abs(q) > eps)
    tau_f_0 = tau_b_f_0*sign(q);
else
    tau_f_0 = 0;
end

if (abs(m) > eps)
    tau_f_1 = tau_b_f_1*sign(m);
else
    tau_f_1 = 0;
end

if (model == 1)
    q_dot = (1/b)*(d*r - tau_f_0 - a_a*q - c*sin(p));
    m_dot = 0;
else
    q_dot =  -(tau_f_0*z_z + b_b*q*z_z - p_p*r*z_z + a*d_d^2*tau_f_0 - f*t*t_t*z_z + a*e^2*tau_f_0*sin(p)^2 + a*b_b*d_d^2*q - a*d_d^2*p_p*r + a^2*e^3*g*sin(p)^3 + a^2*d_d^2*e*g*sin(p) + a*b_b*e^2*q*sin(p)^2 - a*e^2*p_p*r*sin(p)^2 - a^2*e^4*m^2*cos(p)*sin(p)^3 + a*d_d*e*tau_f_1*cos(p) - a*d_d^2*f*t*t_t + a*e*g*z_z*sin(p) - a*e^2*f*t*t_t*sin(p)^2 - a^2*d_d^2*e^2*m^2*cos(p)*sin(p) + a*c_c*d_d*e*m*cos(p) + a^2*d_d^2*e^2*q^2*cos(p)*sin(p) - a*d_d*e*t*t_t*cos(p) - a*e^2*m^2*z_z*cos(p)*sin(p) + 2*a^2*d_d*e^3*m*q*cos(p)^2*sin(p) - a*d_d*e*f*p_p*r*cos(p))/(- a^2*d_d^2*e^2*cos(p)^2 + a^2*d_d^2*e^2 + a^2*e^4*sin(p)^2 + y_y*a*d_d^2 + y_y*a*e^2*sin(p)^2 + z_z*a*e^2 + y_y*z_z);
    m_dot = -(tau_f_1*y_y + c_c*m*y_y - t*t_t*y_y + a*e^2*tau_f_1 - f*p_p*r*y_y + a*c_c*e^2*m - a*e^2*t*t_t - a*e^2*f*p_p*r + a*d_d*e*tau_f_0*cos(p) + a^2*d_d*e^3*q^2*sin(p) - a^2*d_d*e^3*m^2*cos(p)^2*sin(p) + a*b_b*d_d*e*q*cos(p) - a*d_d*e*p_p*r*cos(p) + a^2*d_d*e^2*g*cos(p)*sin(p) + 2*a^2*e^4*m*q*cos(p)*sin(p) + a*d_d*e*q^2*y_y*sin(p) + 2*a*e^2*m*q*y_y*cos(p)*sin(p) - a*d_d*e*f*t*t_t*cos(p))/(- a^2*d_d^2*e^2*cos(p)^2 + a^2*d_d^2*e^2 + a^2*e^4*sin(p)^2 + y_y*a*d_d^2 + y_y*a*e^2*sin(p)^2 + z_z*a*e^2 + y_y*z_z);
end

x_dot = [q; q_dot; m; m_dot];

end

== matlab function Quanser_AERO_Simulation_2020b/Quanser AERO/Quanser AERO System Dynamics/MATLAB Function ==
  data: x input; u input; x_dot output; model input; a parameter; b parameter; c parameter; d parameter; e parameter; f parameter; g parameter; a_a parameter; b_b parameter; c_c parameter; d_d parameter; p_p parameter; t_t parameter; y_y parameter; z_z parameter
% ============================================================= %
%    This function computes the dynamics for the Quanser AERO   %
%    It takes the current input u = (V0, V1), the current       %
%    state x = (theta, theta_dot, psi, psi_dot) and the model   %
%    configuration ("1DOF": 1 or "2DOF": 2) and outputs x_dot   %
%    Created by Vincent Liu (liuv2@student.unimelb.edu.au)      %
%    For ELEN90064 Advanced Control Systems Workshops           %
%    Last updated: 29-07-21                                     %
% ============================================================= %

function x_dot = get_x_dot(x, u, model, a, b, c, d, e, f, g, a_a, b_b, c_c, d_d, p_p, t_t, y_y, z_z)

if (model == 1)
    tau_b_f_0 = 0.8*d;
else
    tau_b_f_0 = 0.8*p_p;
end
tau_b_f_1 = t_t;

eps = 1e-8;

p = x(1); q = x(2); n = x(3); m = x(4);
r = u(1); t = u(2);

q_dot = 0.0;
m_dot = 0.0;
tau_f_0 = 0;

if (abs(q) > eps)
    tau_f_0 = tau_b_f_0*sign(q);
else
    tau_f_0 = 0;
end

if (abs(m) > eps)
    tau_f_1 = tau_b_f_1*sign(m);
else
    tau_f_1 = 0;
end

if (model == 1)
    q_dot = (1/b)*(d*r - tau_f_0 - a_a*q - c*sin(p));
    m_dot = 0;
else
    q_dot =  -(tau_f_0*z_z + b_b*q*z_z - p_p*r*z_z + a*d_d^2*tau_f_0 - f*t*t_t*z_z + a*e^2*tau_f_0*sin(p)^2 + a*b_b*d_d^2*q - a*d_d^2*p_p*r + a^2*e^3*g*sin(p)^3 + a^2*d_d^2*e*g*sin(p) + a*b_b*e^2*q*sin(p)^2 - a*e^2*p_p*r*sin(p)^2 - a^2*e^4*m^2*cos(p)*sin(p)^3 + a*d_d*e*tau_f_1*cos(p) - a*d_d^2*f*t*t_t + a*e*g*z_z*sin(p) - a*e^2*f*t*t_t*sin(p)^2 - a^2*d_d^2*e^2*m^2*cos(p)*sin(p) + a*c_c*d_d*e*m*cos(p) + a^2*d_d^2*e^2*q^2*cos(p)*sin(p) - a*d_d*e*t*t_t*cos(p) - a*e^2*m^2*z_z*cos(p)*sin(p) + 2*a^2*d_d*e^3*m*q*cos(p)^2*sin(p) - a*d_d*e*f*p_p*r*cos(p))/(- a^2*d_d^2*e^2*cos(p)^2 + a^2*d_d^2*e^2 + a^2*e^4*sin(p)^2 + y_y*a*d_d^2 + y_y*a*e^2*sin(p)^2 + z_z*a*e^2 + y_y*z_z);
    m_dot = -(tau_f_1*y_y + c_c*m*y_y - t*t_t*y_y + a*e^2*tau_f_1 - f*p_p*r*y_y + a*c_c*e^2*m - a*e^2*t*t_t - a*e^2*f*p_p*r + a*d_d*e*tau_f_0*cos(p) + a^2*d_d*e^3*q^2*sin(p) - a^2*d_d*e^3*m^2*cos(p)^2*sin(p) + a*b_b*d_d*e*q*cos(p) - a*d_d*e*p_p*r*cos(p) + a^2*d_d*e^2*g*cos(p)*sin(p) + 2*a^2*e^4*m*q*cos(p)*sin(p) + a*d_d*e*q^2*y_y*sin(p) + 2*a*e^2*m*q*y_y*cos(p)*sin(p) - a*d_d*e*f*t*t_t*cos(p))/(- a^2*d_d^2*e^2*cos(p)^2 + a^2*d_d^2*e^2 + a^2*e^4*sin(p)^2 + y_y*a*d_d^2 + y_y*a*e^2*sin(p)^2 + z_z*a*e^2 + y_y*z_z);
end

x_dot = [q; q_dot; m; m_dot];

end

== matlab function Quanser_AERO_Simulation_2020b/Quanser AERO3/Quanser AERO System Dynamics/MATLAB Function ==
  data: x input; u input; x_dot output; model input; a parameter; b parameter; c parameter; d parameter; e parameter; f parameter; g parameter; a_a parameter; b_b parameter; c_c parameter; d_d parameter; p_p parameter; t_t parameter; y_y parameter; z_z parameter
% ============================================================= %
%    This function computes the dynamics for the Quanser AERO   %
%    It takes the current input u = (V0, V1), the current       %
%    state x = (theta, theta_dot, psi, psi_dot) and the model   %
%    configuration ("1DOF": 1 or "2DOF": 2) and outputs x_dot   %
%    Created by Vincent Liu (liuv2@student.unimelb.edu.au)      %
%    For ELEN90064 Advanced Control Systems Workshops           %
%    Last updated: 29-07-21                                     %
% ============================================================= %

function x_dot = get_x_dot(x, u, model, a, b, c, d, e, f, g, a_a, b_b, c_c, d_d, p_p, t_t, y_y, z_z)

if (model == 1)
    tau_b_f_0 = 0.8*d;
else
    tau_b_f_0 = 0.8*p_p;
end
tau_b_f_1 = t_t;

eps = 1e-8;

p = x(1); q = x(2); n = x(3); m = x(4);
r = u(1); t = u(2);

q_dot = 0.0;
m_dot = 0.0;
tau_f_0 = 0;

if (abs(q) > eps)
    tau_f_0 = tau_b_f_0*sign(q);
else
    tau_f_0 = 0;
end

if (abs(m) > eps)
    tau_f_1 = tau_b_f_1*sign(m);
else
    tau_f_1 = 0;
end

if (model == 1)
    q_dot = (1/b)*(d*r - tau_f_0 - a_a*q - c*sin(p));
    m_dot = 0;
else
    q_dot =  -(tau_f_0*z_z + b_b*q*z_z - p_p*r*z_z + a*d_d^2*tau_f_0 - f*t*t_t*z_z + a*e^2*tau_f_0*sin(p)^2 + a*b_b*d_d^2*q - a*d_d^2*p_p*r + a^2*e^3*g*sin(p)^3 + a^2*d_d^2*e*g*sin(p) + a*b_b*e^2*q*sin(p)^2 - a*e^2*p_p*r*sin(p)^2 - a^2*e^4*m^2*cos(p)*sin(p)^3 + a*d_d*e*tau_f_1*cos(p) - a*d_d^2*f*t*t_t + a*e*g*z_z*sin(p) - a*e^2*f*t*t_t*sin(p)^2 - a^2*d_d^2*e^2*m^2*cos(p)*sin(p) + a*c_c*d_d*e*m*cos(p) + a^2*d_d^2*e^2*q^2*cos(p)*sin(p) - a*d_d*e*t*t_t*cos(p) - a*e^2*m^2*z_z*cos(p)*sin(p) + 2*a^2*d_d*e^3*m*q*cos(p)^2*sin(p) - a*d_d*e*f*p_p*r*cos(p))/(- a^2*d_d^2*e^2*cos(p)^2 + a^2*d_d^2*e^2 + a^2*e^4*sin(p)^2 + y_y*a*d_d^2 + y_y*a*e^2*sin(p)^2 + z_z*a*e^2 + y_y*z_z);
    m_dot = -(tau_f_1*y_y + c_c*m*y_y - t*t_t*y_y + a*e^2*tau_f_1 - f*p_p*r*y_y + a*c_c*e^2*m - a*e^2*t*t_t - a*e^2*f*p_p*r + a*d_d*e*tau_f_0*cos(p) + a^2*d_d*e^3*q^2*sin(p) - a^2*d_d*e^3*m^2*cos(p)^2*sin(p) + a*b_b*d_d*e*q*cos(p) - a*d_d*e*p_p*r*cos(p) + a^2*d_d*e^2*g*cos(p)*sin(p) + 2*a^2*e^4*m*q*cos(p)*sin(p) + a*d_d*e*q^2*y_y*sin(p) + 2*a*e^2*m*q*y_y*cos(p)*sin(p) - a*d_d*e*f*t*t_t*cos(p))/(- a^2*d_d^2*e^2*cos(p)^2 + a^2*d_d^2*e^2 + a^2*e^4*sin(p)^2 + y_y*a*d_d^2 + y_y*a*e^2*sin(p)^2 + z_z*a*e^2 + y_y*z_z);
end

x_dot = [q; q_dot; m; m_dot];

end

== matlab function Quanser_AERO_Simulation_2020b/Quanser AERO4/Quanser AERO System Dynamics/MATLAB Function ==
  data: x input; u input; x_dot output; model input; a parameter; b parameter; c parameter; d parameter; e parameter; f parameter; g parameter; a_a parameter; b_b parameter; c_c parameter; d_d parameter; p_p parameter; t_t parameter; y_y parameter; z_z parameter
% ============================================================= %
%    This function computes the dynamics for the Quanser AERO   %
%    It takes the current input u = (V0, V1), the current       %
%    state x = (theta, theta_dot, psi, psi_dot) and the model   %
%    configuration ("1DOF": 1 or "2DOF": 2) and outputs x_dot   %
%    Created by Vincent Liu (liuv2@student.unimelb.edu.au)      %
%    For ELEN90064 Advanced Control Systems Workshops           %
%    Last updated: 29-07-21                                     %
% ============================================================= %

function x_dot = get_x_dot(x, u, model, a, b, c, d, e, f, g, a_a, b_b, c_c, d_d, p_p, t_t, y_y, z_z)

if (model == 1)
    tau_b_f_0 = 0.8*d;
else
    tau_b_f_0 = 0.8*p_p;
end
tau_b_f_1 = t_t;

eps = 1e-8;

p = x(1); q = x(2); n = x(3); m = x(4);
r = u(1); t = u(2);

q_dot = 0.0;
m_dot = 0.0;
tau_f_0 = 0;

if (abs(q) > eps)
    tau_f_0 = tau_b_f_0*sign(q);
else
    tau_f_0 = 0;
end

if (abs(m) > eps)
    tau_f_1 = tau_b_f_1*sign(m);
else
    tau_f_1 = 0;
end

if (model == 1)
    q_dot = (1/b)*(d*r - tau_f_0 - a_a*q - c*sin(p));
    m_dot = 0;
else
    q_dot =  -(tau_f_0*z_z + b_b*q*z_z - p_p*r*z_z + a*d_d^2*tau_f_0 - f*t*t_t*z_z + a*e^2*tau_f_0*sin(p)^2 + a*b_b*d_d^2*q - a*d_d^2*p_p*r + a^2*e^3*g*sin(p)^3 + a^2*d_d^2*e*g*sin(p) + a*b_b*e^2*q*sin(p)^2 - a*e^2*p_p*r*sin(p)^2 - a^2*e^4*m^2*cos(p)*sin(p)^3 + a*d_d*e*tau_f_1*cos(p) - a*d_d^2*f*t*t_t + a*e*g*z_z*sin(p) - a*e^2*f*t*t_t*sin(p)^2 - a^2*d_d^2*e^2*m^2*cos(p)*sin(p) + a*c_c*d_d*e*m*cos(p) + a^2*d_d^2*e^2*q^2*cos(p)*sin(p) - a*d_d*e*t*t_t*cos(p) - a*e^2*m^2*z_z*cos(p)*sin(p) + 2*a^2*d_d*e^3*m*q*cos(p)^2*sin(p) - a*d_d*e*f*p_p*r*cos(p))/(- a^2*d_d^2*e^2*cos(p)^2 + a^2*d_d^2*e^2 + a^2*e^4*sin(p)^2 + y_y*a*d_d^2 + y_y*a*e^2*sin(p)^2 + z_z*a*e^2 + y_y*z_z);
    m_dot = -(tau_f_1*y_y + c_c*m*y_y - t*t_t*y_y + a*e^2*tau_f_1 - f*p_p*r*y_y + a*c_c*e^2*m - a*e^2*t*t_t - a*e^2*f*p_p*r + a*d_d*e*tau_f_0*cos(p) + a^2*d_d*e^3*q^2*sin(p) - a^2*d_d*e^3*m^2*cos(p)^2*sin(p) + a*b_b*d_d*e*q*cos(p) - a*d_d*e*p_p*r*cos(p) + a^2*d_d*e^2*g*cos(p)*sin(p) + 2*a^2*e^4*m*q*cos(p)*sin(p) + a*d_d*e*q^2*y_y*sin(p) + 2*a*e^2*m*q*y_y*cos(p)*sin(p) - a*d_d*e*f*t*t_t*cos(p))/(- a^2*d_d^2*e^2*cos(p)^2 + a^2*d_d^2*e^2 + a^2*e^4*sin(p)^2 + y_y*a*d_d^2 + y_y*a*e^2*sin(p)^2 + z_z*a*e^2 + y_y*z_z);
end

x_dot = [q; q_dot; m; m_dot];

end
